simulink model "prac_4_rodillo_simulink"  (R2025a)
settings: Solver=VariableStepAuto  StartTime=0.0  StopTime=10.0  RelTol=1e-3
InitFcn:
  | m=10;
  | k=100;
  | r=0.05;
settings Model: Creator=USER  LastModifiedBy=USER

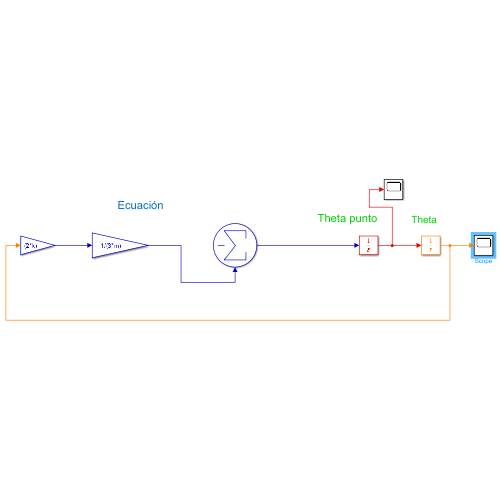
[thumbnail: Simulink's stored preview of the top-level diagram]
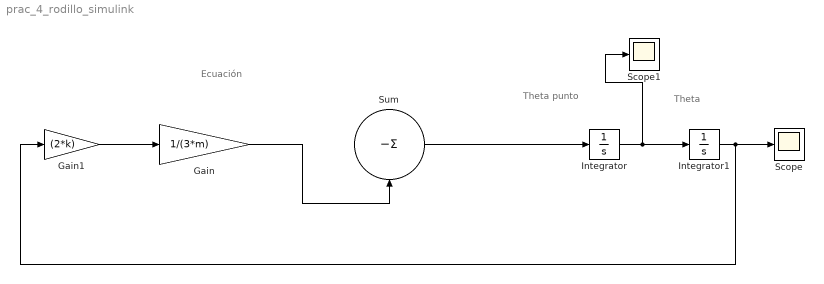
== system prac_4_rodillo_simulink ==
  note: Ecuación
  note: Theta punto
  note: Theta
  Gain : Gain  Gain=1/(3*m)
  Gain1 : Gain  Gain=(2*k)
  Integrator : Integrator
  Integrator1 : Integrator  InitialCondition=2
  Scope : Scope
      settings: ActiveDisplayYMinimum=-2.4992814333514262  ActiveDisplayYMaximum=2.4999201592612694
  Scope1 : Scope
      settings: ActiveDisplayYMinimum=-6.4491368232872706  ActiveDisplayYMaximum=6.4538718436924905
  Sum : Sum  Inputs=|-
  wires:
  Integrator1/1 -> Scope/1, Gain1/1
  Integrator/1 -> Scope1/1, Integrator1/1
  Gain/1 -> Sum/1
  Sum/1 -> Integrator/1
  Gain1/1 -> Gain/1
